simulink model "canTransceiverModel"  (R2018a)
settings: Solver=FixedStepDiscrete  StartTime=0.0  StopTime=50  RelTol=1e-3  EnableMultiTasking=on
values from neighbouring files (symbols this model uses):
  sampleTime = 0.040    (= 0.04)    [canTrasceiverConfig.m]
  sensorLocationConfig = uint8(sensorLocationConfig)    [canTrasceiverConfig.m]
undefined symbols (not defined in the file or in its folder): canChannel, CRC
libraries: simulink x81, canmsglib x27, canlib x8, commcrc2 x1
(part 2 of 5)

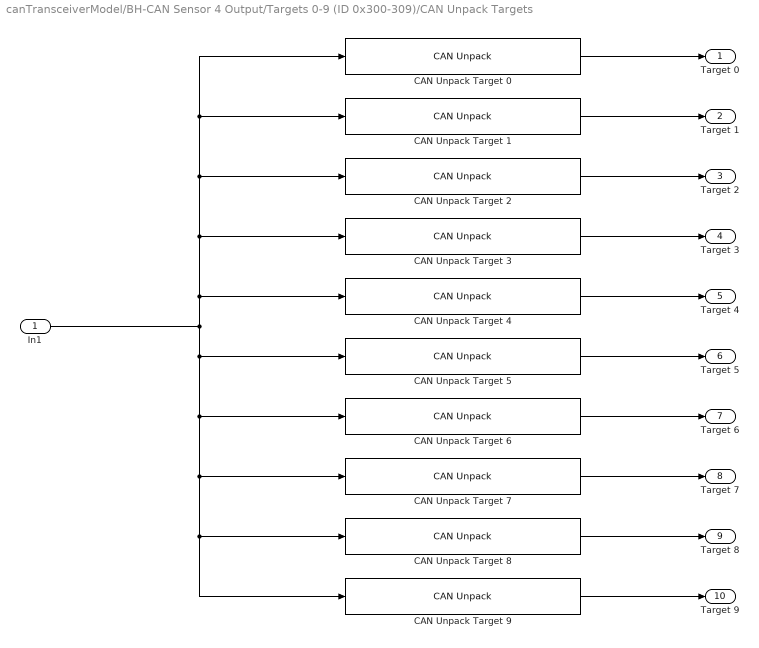
== system canTransceiverModel/BH-CAN Sensor 4 Output/Targets 0-9 (ID 0x300-309)/CAN Unpack Targets ==
  In1 : Inport
  CAN Unpack Target 0 : canmsglib/CAN Unpack  CANdbFile=VehicleInfo.dbc  MsgList=WheelSpeeds  MsgName=Target 0  MsgIDType=Standard (11-bit identifier)  MsgIdentifier=hex2dec('300')  MsgLength=8  SignalInfo=LF_WSpeed$8$16$2$2$1$0$1.000000e-02$-100$0$2000$#LR_WSpeed$40$16$2$2$1$0$1.000000e-02$-100$0$2000$#RF_WSpeed$24$16$2$2$1$0$1.000000e-02$-100$0$2000$#RR_WSpeed$56$16$2$2$1$0$1.000000e-02$-100$0$2000$#  NSignals=4  IDPort=off  TimestampPort=off  ErrorPort=off  RemotePort=off  LengthPort=off  StatusPort=off  StartBits=str2num('[int32(8);int32(40);int32(24);int32(56)]')  SignalSizes=str2num('[int32(16);int32(16);int32(16);int32(16)]')  ByteOrders=str2num('[int32(2);int32(2);int32(2);int32(2)]')  DataTypes=str2num('[int32(2);int32(2);int32(2);int32(2)]')  MultiplexTypes=str2num('[int32(1);int32(1);int32(1);int32(1)]')  MultiplexValues=str2num('[double(0);double(0);double(0);double(0)]')  Factors=str2num('[double(1.000000e-02);double(1.000000e-02);double(1.000000e-02);double(1.000000e-02)]')  Offsets=str2num('[double(-100);double(-100);double(-100);double(-100)]')  Minimums=str2num('[double(0);double(0);double(0);double(0)]')  Maximums=str2num('[double(2000);double(2000);double(2000);double(2000)]')  ApplyMinMax=off
      settings: SourceProductName=Simulink Real-Time  SourceProductBaseCode=XP  DataFormat=raw data
  CAN Unpack Target 1 : canmsglib/CAN Unpack  CANdbFile=VehicleInfo.dbc  MsgList=WheelSpeeds  MsgName=Target 1  MsgIDType=Standard (11-bit identifier)  MsgIdentifier=hex2dec('301')  MsgLength=8  SignalInfo=LF_WSpeed$8$16$2$2$1$0$1.000000e-02$-100$0$2000$#LR_WSpeed$40$16$2$2$1$0$1.000000e-02$-100$0$2000$#RF_WSpeed$24$16$2$2$1$0$1.000000e-02$-100$0$2000$#RR_WSpeed$56$16$2$2$1$0$1.000000e-02$-100$0$2000$#  NSignals=4  IDPort=off  TimestampPort=off  ErrorPort=off  RemotePort=off  LengthPort=off  StatusPort=off  StartBits=str2num('[int32(8);int32(40);int32(24);int32(56)]')  SignalSizes=str2num('[int32(16);int32(16);int32(16);int32(16)]')  ByteOrders=str2num('[int32(2);int32(2);int32(2);int32(2)]')  DataTypes=str2num('[int32(2);int32(2);int32(2);int32(2)]')  MultiplexTypes=str2num('[int32(1);int32(1);int32(1);int32(1)]')  MultiplexValues=str2num('[double(0);double(0);double(0);double(0)]')  Factors=str2num('[double(1.000000e-02);double(1.000000e-02);double(1.000000e-02);double(1.000000e-02)]')  Offsets=str2num('[double(-100);double(-100);double(-100);double(-100)]')  Minimums=str2num('[double(0);double(0);double(0);double(0)]')  Maximums=str2num('[double(2000);double(2000);double(2000);double(2000)]')  ApplyMinMax=off
      settings: SourceProductName=Simulink Real-Time  SourceProductBaseCode=XP  DataFormat=raw data
  CAN Unpack Target 2 : canmsglib/CAN Unpack  CANdbFile=VehicleInfo.dbc  MsgList=WheelSpeeds  MsgName=Target 2  MsgIDType=Standard (11-bit identifier)  MsgIdentifier=hex2dec('302')  MsgLength=8  SignalInfo=LF_WSpeed$8$16$2$2$1$0$1.000000e-02$-100$0$2000$#LR_WSpeed$40$16$2$2$1$0$1.000000e-02$-100$0$2000$#RF_WSpeed$24$16$2$2$1$0$1.000000e-02$-100$0$2000$#RR_WSpeed$56$16$2$2$1$0$1.000000e-02$-100$0$2000$#  NSignals=4  IDPort=off  TimestampPort=off  ErrorPort=off  RemotePort=off  LengthPort=off  StatusPort=off  StartBits=str2num('[int32(8);int32(40);int32(24);int32(56)]')  SignalSizes=str2num('[int32(16);int32(16);int32(16);int32(16)]')  ByteOrders=str2num('[int32(2);int32(2);int32(2);int32(2)]')  DataTypes=str2num('[int32(2);int32(2);int32(2);int32(2)]')  MultiplexTypes=str2num('[int32(1);int32(1);int32(1);int32(1)]')  MultiplexValues=str2num('[double(0);double(0);double(0);double(0)]')  Factors=str2num('[double(1.000000e-02);double(1.000000e-02);double(1.000000e-02);double(1.000000e-02)]')  Offsets=str2num('[double(-100);double(-100);double(-100);double(-100)]')  Minimums=str2num('[double(0);double(0);double(0);double(0)]')  Maximums=str2num('[double(2000);double(2000);double(2000);double(2000)]')  ApplyMinMax=off
      settings: SourceProductName=Simulink Real-Time  SourceProductBaseCode=XP  DataFormat=raw data
  CAN Unpack Target 3 : canmsglib/CAN Unpack  CANdbFile=VehicleInfo.dbc  MsgList=WheelSpeeds  MsgName=Target 3  MsgIDType=Standard (11-bit identifier)  MsgIdentifier=hex2dec('303')  MsgLength=8  SignalInfo=LF_WSpeed$8$16$2$2$1$0$1.000000e-02$-100$0$2000$#LR_WSpeed$40$16$2$2$1$0$1.000000e-02$-100$0$2000$#RF_WSpeed$24$16$2$2$1$0$1.000000e-02$-100$0$2000$#RR_WSpeed$56$16$2$2$1$0$1.000000e-02$-100$0$2000$#  NSignals=4  IDPort=off  TimestampPort=off  ErrorPort=off  RemotePort=off  LengthPort=off  StatusPort=off  StartBits=str2num('[int32(8);int32(40);int32(24);int32(56)]')  SignalSizes=str2num('[int32(16);int32(16);int32(16);int32(16)]')  ByteOrders=str2num('[int32(2);int32(2);int32(2);int32(2)]')  DataTypes=str2num('[int32(2);int32(2);int32(2);int32(2)]')  MultiplexTypes=str2num('[int32(1);int32(1);int32(1);int32(1)]')  MultiplexValues=str2num('[double(0);double(0);double(0);double(0)]')  Factors=str2num('[double(1.000000e-02);double(1.000000e-02);double(1.000000e-02);double(1.000000e-02)]')  Offsets=str2num('[double(-100);double(-100);double(-100);double(-100)]')  Minimums=str2num('[double(0);double(0);double(0);double(0)]')  Maximums=str2num('[double(2000);double(2000);double(2000);double(2000)]')  ApplyMinMax=off
      settings: SourceProductName=Simulink Real-Time  SourceProductBaseCode=XP  DataFormat=raw data
  CAN Unpack Target 4 : canmsglib/CAN Unpack  CANdbFile=VehicleInfo.dbc  MsgList=WheelSpeeds  MsgName=Target 4  MsgIDType=Standard (11-bit identifier)  MsgIdentifier=hex2dec('304')  MsgLength=8  SignalInfo=LF_WSpeed$8$16$2$2$1$0$1.000000e-02$-100$0$2000$#LR_WSpeed$40$16$2$2$1$0$1.000000e-02$-100$0$2000$#RF_WSpeed$24$16$2$2$1$0$1.000000e-02$-100$0$2000$#RR_WSpeed$56$16$2$2$1$0$1.000000e-02$-100$0$2000$#  NSignals=4  IDPort=off  TimestampPort=off  ErrorPort=off  RemotePort=off  LengthPort=off  StatusPort=off  StartBits=str2num('[int32(8);int32(40);int32(24);int32(56)]')  SignalSizes=str2num('[int32(16);int32(16);int32(16);int32(16)]')  ByteOrders=str2num('[int32(2);int32(2);int32(2);int32(2)]')  DataTypes=str2num('[int32(2);int32(2);int32(2);int32(2)]')  MultiplexTypes=str2num('[int32(1);int32(1);int32(1);int32(1)]')  MultiplexValues=str2num('[double(0);double(0);double(0);double(0)]')  Factors=str2num('[double(1.000000e-02);double(1.000000e-02);double(1.000000e-02);double(1.000000e-02)]')  Offsets=str2num('[double(-100);double(-100);double(-100);double(-100)]')  Minimums=str2num('[double(0);double(0);double(0);double(0)]')  Maximums=str2num('[double(2000);double(2000);double(2000);double(2000)]')  ApplyMinMax=off
      settings: SourceProductName=Simulink Real-Time  SourceProductBaseCode=XP  DataFormat=raw data
  CAN Unpack Target 5 : canmsglib/CAN Unpack  CANdbFile=VehicleInfo.dbc  MsgList=WheelSpeeds  MsgName=Target 5  MsgIDType=Standard (11-bit identifier)  MsgIdentifier=hex2dec('305')  MsgLength=8  SignalInfo=LF_WSpeed$8$16$2$2$1$0$1.000000e-02$-100$0$2000$#LR_WSpeed$40$16$2$2$1$0$1.000000e-02$-100$0$2000$#RF_WSpeed$24$16$2$2$1$0$1.000000e-02$-100$0$2000$#RR_WSpeed$56$16$2$2$1$0$1.000000e-02$-100$0$2000$#  NSignals=4  IDPort=off  TimestampPort=off  ErrorPort=off  RemotePort=off  LengthPort=off  StatusPort=off  StartBits=str2num('[int32(8);int32(40);int32(24);int32(56)]')  SignalSizes=str2num('[int32(16);int32(16);int32(16);int32(16)]')  ByteOrders=str2num('[int32(2);int32(2);int32(2);int32(2)]')  DataTypes=str2num('[int32(2);int32(2);int32(2);int32(2)]')  MultiplexTypes=str2num('[int32(1);int32(1);int32(1);int32(1)]')  MultiplexValues=str2num('[double(0);double(0);double(0);double(0)]')  Factors=str2num('[double(1.000000e-02);double(1.000000e-02);double(1.000000e-02);double(1.000000e-02)]')  Offsets=str2num('[double(-100);double(-100);double(-100);double(-100)]')  Minimums=str2num('[double(0);double(0);double(0);double(0)]')  Maximums=str2num('[double(2000);double(2000);double(2000);double(2000)]')  ApplyMinMax=off
      settings: SourceProductName=Simulink Real-Time  SourceProductBaseCode=XP  DataFormat=raw data
  CAN Unpack Target 6 : canmsglib/CAN Unpack  CANdbFile=VehicleInfo.dbc  MsgList=WheelSpeeds  MsgName=Target 6  MsgIDType=Standard (11-bit identifier)  MsgIdentifier=hex2dec('306')  MsgLength=8  SignalInfo=LF_WSpeed$8$16$2$2$1$0$1.000000e-02$-100$0$2000$#LR_WSpeed$40$16$2$2$1$0$1.000000e-02$-100$0$2000$#RF_WSpeed$24$16$2$2$1$0$1.000000e-02$-100$0$2000$#RR_WSpeed$56$16$2$2$1$0$1.000000e-02$-100$0$2000$#  NSignals=4  IDPort=off  TimestampPort=off  ErrorPort=off  RemotePort=off  LengthPort=off  StatusPort=off  StartBits=str2num('[int32(8);int32(40);int32(24);int32(56)]')  SignalSizes=str2num('[int32(16);int32(16);int32(16);int32(16)]')  ByteOrders=str2num('[int32(2);int32(2);int32(2);int32(2)]')  DataTypes=str2num('[int32(2);int32(2);int32(2);int32(2)]')  MultiplexTypes=str2num('[int32(1);int32(1);int32(1);int32(1)]')  MultiplexValues=str2num('[double(0);double(0);double(0);double(0)]')  Factors=str2num('[double(1.000000e-02);double(1.000000e-02);double(1.000000e-02);double(1.000000e-02)]')  Offsets=str2num('[double(-100);double(-100);double(-100);double(-100)]')  Minimums=str2num('[double(0);double(0);double(0);double(0)]')  Maximums=str2num('[double(2000);double(2000);double(2000);double(2000)]')  ApplyMinMax=off
      settings: SourceProductName=Simulink Real-Time  SourceProductBaseCode=XP  DataFormat=raw data
  CAN Unpack Target 7 : canmsglib/CAN Unpack  CANdbFile=VehicleInfo.dbc  MsgList=WheelSpeeds  MsgName=Target 7  MsgIDType=Standard (11-bit identifier)  MsgIdentifier=hex2dec('307')  MsgLength=8  SignalInfo=LF_WSpeed$8$16$2$2$1$0$1.000000e-02$-100$0$2000$#LR_WSpeed$40$16$2$2$1$0$1.000000e-02$-100$0$2000$#RF_WSpeed$24$16$2$2$1$0$1.000000e-02$-100$0$2000$#RR_WSpeed$56$16$2$2$1$0$1.000000e-02$-100$0$2000$#  NSignals=4  IDPort=off  TimestampPort=off  ErrorPort=off  RemotePort=off  LengthPort=off  StatusPort=off  StartBits=str2num('[int32(8);int32(40);int32(24);int32(56)]')  SignalSizes=str2num('[int32(16);int32(16);int32(16);int32(16)]')  ByteOrders=str2num('[int32(2);int32(2);int32(2);int32(2)]')  DataTypes=str2num('[int32(2);int32(2);int32(2);int32(2)]')  MultiplexTypes=str2num('[int32(1);int32(1);int32(1);int32(1)]')  MultiplexValues=str2num('[double(0);double(0);double(0);double(0)]')  Factors=str2num('[double(1.000000e-02);double(1.000000e-02);double(1.000000e-02);double(1.000000e-02)]')  Offsets=str2num('[double(-100);double(-100);double(-100);double(-100)]')  Minimums=str2num('[double(0);double(0);double(0);double(0)]')  Maximums=str2num('[double(2000);double(2000);double(2000);double(2000)]')  ApplyMinMax=off
      settings: SourceProductName=Simulink Real-Time  SourceProductBaseCode=XP  DataFormat=raw data
  CAN Unpack Target 8 : canmsglib/CAN Unpack  CANdbFile=VehicleInfo.dbc  MsgList=WheelSpeeds  MsgName=Target 8  MsgIDType=Standard (11-bit identifier)  MsgIdentifier=hex2dec('308')  MsgLength=8  SignalInfo=LF_WSpeed$8$16$2$2$1$0$1.000000e-02$-100$0$2000$#LR_WSpeed$40$16$2$2$1$0$1.000000e-02$-100$0$2000$#RF_WSpeed$24$16$2$2$1$0$1.000000e-02$-100$0$2000$#RR_WSpeed$56$16$2$2$1$0$1.000000e-02$-100$0$2000$#  NSignals=4  IDPort=off  TimestampPort=off  ErrorPort=off  RemotePort=off  LengthPort=off  StatusPort=off  StartBits=str2num('[int32(8);int32(40);int32(24);int32(56)]')  SignalSizes=str2num('[int32(16);int32(16);int32(16);int32(16)]')  ByteOrders=str2num('[int32(2);int32(2);int32(2);int32(2)]')  DataTypes=str2num('[int32(2);int32(2);int32(2);int32(2)]')  MultiplexTypes=str2num('[int32(1);int32(1);int32(1);int32(1)]')  MultiplexValues=str2num('[double(0);double(0);double(0);double(0)]')  Factors=str2num('[double(1.000000e-02);double(1.000000e-02);double(1.000000e-02);double(1.000000e-02)]')  Offsets=str2num('[double(-100);double(-100);double(-100);double(-100)]')  Minimums=str2num('[double(0);double(0);double(0);double(0)]')  Maximums=str2num('[double(2000);double(2000);double(2000);double(2000)]')  ApplyMinMax=off
      settings: SourceProductName=Simulink Real-Time  SourceProductBaseCode=XP  DataFormat=raw data
  CAN Unpack Target 9 : canmsglib/CAN Unpack  CANdbFile=VehicleInfo.dbc  MsgList=WheelSpeeds  MsgName=Target 9  MsgIDType=Standard (11-bit identifier)  MsgIdentifier=hex2dec('309')  MsgLength=8  SignalInfo=LF_WSpeed$8$16$2$2$1$0$1.000000e-02$-100$0$2000$#LR_WSpeed$40$16$2$2$1$0$1.000000e-02$-100$0$2000$#RF_WSpeed$24$16$2$2$1$0$1.000000e-02$-100$0$2000$#RR_WSpeed$56$16$2$2$1$0$1.000000e-02$-100$0$2000$#  NSignals=4  IDPort=off  TimestampPort=off  ErrorPort=off  RemotePort=off  LengthPort=off  StatusPort=off  StartBits=str2num('[int32(8);int32(40);int32(24);int32(56)]')  SignalSizes=str2num('[int32(16);int32(16);int32(16);int32(16)]')  ByteOrders=str2num('[int32(2);int32(2);int32(2);int32(2)]')  DataTypes=str2num('[int32(2);int32(2);int32(2);int32(2)]')  MultiplexTypes=str2num('[int32(1);int32(1);int32(1);int32(1)]')  MultiplexValues=str2num('[double(0);double(0);double(0);double(0)]')  Factors=str2num('[double(1.000000e-02);double(1.000000e-02);double(1.000000e-02);double(1.000000e-02)]')  Offsets=str2num('[double(-100);double(-100);double(-100);double(-100)]')  Minimums=str2num('[double(0);double(0);double(0);double(0)]')  Maximums=str2num('[double(2000);double(2000);double(2000);double(2000)]')  ApplyMinMax=off
      settings: SourceProductName=Simulink Real-Time  SourceProductBaseCode=XP  DataFormat=raw data
  Target 0 : Outport
  Target 1 : Outport  Port=2
  Target 2 : Outport  Port=3
  Target 3 : Outport  Port=4
  Target 4 : Outport  Port=5
  Target 5 : Outport  Port=6
  Target 6 : Outport  Port=7
  Target 7 : Outport  Port=8
  Target 8 : Outport  Port=9
  Target 9 : Outport  Port=10
  wires:
  In1/1 -> CAN Unpack Target 0/1, CAN Unpack Target 1/1, CAN Unpack Target 2/1, CAN Unpack Target 3/1, CAN Unpack Target 4/1, CAN Unpack Target 9/1, CAN Unpack Target 8/1, CAN Unpack Target 7/1, CAN Unpack Target 6/1, CAN Unpack Target 5/1
  CAN Unpack Target 3/1 -> Target 3/1
  CAN Unpack Target 8/1 -> Target 8/1
  CAN Unpack Target 2/1 -> Target 2/1
  CAN Unpack Target 1/1 -> Target 1/1
  CAN Unpack Target 4/1 -> Target 4/1
  CAN Unpack Target 5/1 -> Target 5/1
  CAN Unpack Target 7/1 -> Target 7/1
  CAN Unpack Target 6/1 -> Target 6/1
  CAN Unpack Target 0/1 -> Target 0/1
  CAN Unpack Target 9/1 -> Target 9/1

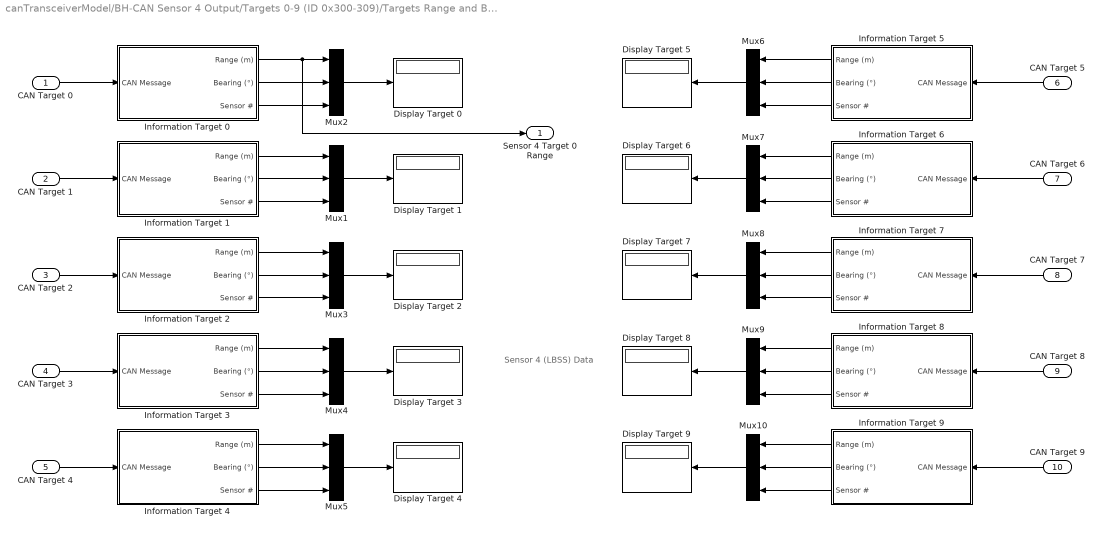
== system canTransceiverModel/BH-CAN Sensor 4 Output/Targets 0-9 (ID 0x300-309)/Targets Range and Bearing Information ==
  note: Sensor 4
      | (LBSS)
      | Data
  CAN Target 0 : Inport
  CAN Target 1 : Inport  Port=2
  CAN Target 2 : Inport  Port=3
  CAN Target 3 : Inport  Port=4
  CAN Target 4 : Inport  Port=5
  CAN Target 5 : Inport  Port=6
  CAN Target 6 : Inport  Port=7
  CAN Target 7 : Inport  Port=8
  CAN Target 8 : Inport  Port=9
  CAN Target 9 : Inport  Port=10
  Display Target {0..9} (10 alike) : Display
  Information Target 0 : Subsystem
  Information Target 1 : Subsystem
  Information Target 2 : Subsystem
  Information Target 3 : Subsystem
  Information Target 4 : Subsystem
  Information Target 5 : Subsystem
  Information Target 6 : Subsystem
  Information Target 7 : Subsystem
  Information Target 8 : Subsystem
  Information Target 9 : Subsystem
  Mux{1..10} (10 alike) : Mux  Inputs=3
  Sensor 4 Target 0 Range : Outport
  wires:
  Information Target 0/2(Bearing (°)) -> Mux2/2
  CAN Target 0/1 -> Information Target 0/1(CAN Message)
  Information Target 0/3(Sensor #) -> Mux2/3
  CAN Target 1/1 -> Information Target 1/1(CAN Message)
  Information Target 1/1(Range (m)) -> Mux1/1
  Information Target 1/3(Sensor #) -> Mux1/3
  Information Target 1/2(Bearing (°)) -> Mux1/2
  CAN Target 2/1 -> Information Target 2/1(CAN Message)
  Information Target 2/1(Range (m)) -> Mux3/1
  Information Target 2/3(Sensor #) -> Mux3/3
  Information Target 2/2(Bearing (°)) -> Mux3/2
  CAN Target 3/1 -> Information Target 3/1(CAN Message)
  Information Target 3/1(Range (m)) -> Mux4/1
  Information Target 3/3(Sensor #) -> Mux4/3
  Information Target 3/2(Bearing (°)) -> Mux4/2
  CAN Target 4/1 -> Information Target 4/1(CAN Message)
  Information Target 4/1(Range (m)) -> Mux5/1
  Information Target 4/3(Sensor #) -> Mux5/3
  Mux5/1 -> Display Target 4/1
  Information Target 4/2(Bearing (°)) -> Mux5/2
  CAN Target 5/1 -> Information Target 5/1(CAN Message)
  Information Target 5/1(Range (m)) -> Mux6/1
  Information Target 5/3(Sensor #) -> Mux6/3
  Mux6/1 -> Display Target 5/1
  Information Target 5/2(Bearing (°)) -> Mux6/2
  Information Target 6/2(Bearing (°)) -> Mux7/2
  Mux7/1 -> Display Target 6/1
  Information Target 6/3(Sensor #) -> Mux7/3
  CAN Target 6/1 -> Information Target 6/1(CAN Message)
  Information Target 6/1(Range (m)) -> Mux7/1
  Information Target 7/2(Bearing (°)) -> Mux8/2
  Mux8/1 -> Display Target 7/1
  Information Target 7/3(Sensor #) -> Mux8/3
  CAN Target 7/1 -> Information Target 7/1(CAN Message)
  Information Target 7/1(Range (m)) -> Mux8/1
  Information Target 8/2(Bearing (°)) -> Mux9/2
  Mux9/1 -> Display Target 8/1
  Information Target 8/3(Sensor #) -> Mux9/3
  CAN Target 8/1 -> Information Target 8/1(CAN Message)
  Information Target 8/1(Range (m)) -> Mux9/1
  Information Target 9/2(Bearing (°)) -> Mux10/2
  Mux10/1 -> Display Target 9/1
  Information Target 9/3(Sensor #) -> Mux10/3
  CAN Target 9/1 -> Information Target 9/1(CAN Message)
  Information Target 9/1(Range (m)) -> Mux10/1
  Mux2/1 -> Display Target 0/1
  Mux4/1 -> Display Target 3/1
  Mux1/1 -> Display Target 1/1
  Mux3/1 -> Display Target 2/1
  Information Target 0/1(Range (m)) -> Sensor 4 Target 0 Range/1, Mux2/1

== system canTransceiverModel/BH-CAN Sensor 3 Output/Targets 0-9 (ID 0x300-309)/Targets Range and Bearing Information/Information Target 0 ==
  CAN Message : Inport
  Check Target Format : Subsystem
  Target Format 2 : Subsystem
  Terminator : Terminator
  Terminator1 : Terminator
  Range (m) : Outport
  Bearing (°) : Outport  Port=2
  Sensor # : Outport  Port=3
  wires:
  Target Format 2/2(Bearing (°)) -> Bearing (°)/1
  CAN Message/1 -> Check Target Format/1(CAN Message), Target Format 2/1(CAN Message)
  Check Target Format/1(Is format 2?) -> Target Format 2/Enable
  Check Target Format/2(Is format 6?) -> Terminator1/1
  Target Format 2/1(Range (m)) -> Range (m)/1
  Target Format 2/3(Sensor #) -> Sensor #/1
  Check Target Format/3(Is neither 2 nor 6?) -> Terminator/1

== system canTransceiverModel/BH-CAN Sensor 3 Output/Targets 0-9 (ID 0x300-309)/Targets Range and Bearing Information/Information Target 1 ==
  CAN Message : Inport
  Check Target Format : Subsystem
  Target Format 2 : Subsystem
  Terminator : Terminator
  Terminator1 : Terminator
  Range (m) : Outport
  Bearing (°) : Outport  Port=2
  Sensor # : Outport  Port=3
  wires:
  Target Format 2/2(Bearing (°)) -> Bearing (°)/1
  CAN Message/1 -> Check Target Format/1(CAN Message), Target Format 2/1(CAN Message)
  Target Format 2/1(Range (m)) -> Range (m)/1
  Target Format 2/3(Sensor #) -> Sensor #/1
  Check Target Format/1(Is format 2?) -> Target Format 2/Enable
  Check Target Format/2(Is format 6?) -> Terminator/1
  Check Target Format/3(Is neither 2 nor 6?) -> Terminator1/1

== system canTransceiverModel/BH-CAN Sensor 3 Output/Targets 0-9 (ID 0x300-309)/Targets Range and Bearing Information/Information Target 2 ==
  CAN Message : Inport
  Check Target Format : Subsystem
  Target Format 2 : Subsystem
  Terminator : Terminator
  Terminator1 : Terminator
  Range (m) : Outport
  Bearing (°) : Outport  Port=2
  Sensor # : Outport  Port=3
  wires:
  Target Format 2/2(Bearing (°)) -> Bearing (°)/1
  CAN Message/1 -> Check Target Format/1(CAN Message), Target Format 2/1(CAN Message)
  Target Format 2/1(Range (m)) -> Range (m)/1
  Target Format 2/3(Sensor #) -> Sensor #/1
  Check Target Format/1(Is format 2?) -> Target Format 2/Enable
  Check Target Format/3(Is neither 2 nor 6?) -> Terminator1/1
  Check Target Format/2(Is format 6?) -> Terminator/1

== system canTransceiverModel/BH-CAN Sensor 3 Output/Targets 0-9 (ID 0x300-309)/Targets Range and Bearing Information/Information Target 3 ==
  CAN Message : Inport
  Check Target Format : Subsystem
  Target Format 2 : Subsystem
  Terminator : Terminator
  Terminator1 : Terminator
  Range (m) : Outport
  Bearing (°) : Outport  Port=2
  Sensor # : Outport  Port=3
  wires:
  Target Format 2/2(Bearing (°)) -> Bearing (°)/1
  CAN Message/1 -> Check Target Format/1(CAN Message), Target Format 2/1(CAN Message)
  Target Format 2/1(Range (m)) -> Range (m)/1
  Target Format 2/3(Sensor #) -> Sensor #/1
  Check Target Format/1(Is format 2?) -> Target Format 2/Enable
  Check Target Format/2(Is format 6?) -> Terminator/1
  Check Target Format/3(Is neither 2 nor 6?) -> Terminator1/1

== system canTransceiverModel/BH-CAN Sensor 3 Output/Targets 0-9 (ID 0x300-309)/Targets Range and Bearing Information/Information Target 4 ==
  CAN Message : Inport
  Check Target Format1 : Subsystem
  Target Format 2 : Subsystem
  Terminator : Terminator
  Terminator1 : Terminator
  Range (m) : Outport
  Bearing (°) : Outport  Port=2
  Sensor # : Outport  Port=3
  wires:
  Target Format 2/2(Bearing (°)) -> Bearing (°)/1
  CAN Message/1 -> Check Target Format1/1(CAN Message), Target Format 2/1(CAN Message)
  Target Format 2/1(Range (m)) -> Range (m)/1
  Target Format 2/3(Sensor #) -> Sensor #/1
  Check Target Format1/1(Is format 2?) -> Target Format 2/Enable
  Check Target Format1/2(Is format 6?) -> Terminator/1
  Check Target Format1/3(Is neither 2 nor 6?) -> Terminator1/1

== system canTransceiverModel/BH-CAN Sensor 3 Output/Targets 0-9 (ID 0x300-309)/Targets Range and Bearing Information/Information Target 5 ==
  CAN Message : Inport
  Check Target Format1 : Subsystem
  Target Format 2 : Subsystem
  Terminator : Terminator
  Terminator1 : Terminator
  Range (m) : Outport
  Bearing (°) : Outport  Port=2
  Sensor # : Outport  Port=3
  wires:
  Target Format 2/2(Bearing (°)) -> Bearing (°)/1
  CAN Message/1 -> Check Target Format1/1(CAN Message), Target Format 2/1(CAN Message)
  Target Format 2/1(Range (m)) -> Range (m)/1
  Target Format 2/3(Sensor #) -> Sensor #/1
  Check Target Format1/1(Is format 2?) -> Target Format 2/Enable
  Check Target Format1/2(Is format 6?) -> Terminator/1
  Check Target Format1/3(Is neither 2 nor 6?) -> Terminator1/1

== system canTransceiverModel/BH-CAN Sensor 3 Output/Targets 0-9 (ID 0x300-309)/Targets Range and Bearing Information/Information Target 6 ==
  CAN Message : Inport
  Check Target Format : Subsystem
  Target Format 2 : Subsystem
  Terminator : Terminator
  Terminator1 : Terminator
  Range (m) : Outport
  Bearing (°) : Outport  Port=2
  Sensor # : Outport  Port=3
  wires:
  Target Format 2/2(Bearing (°)) -> Bearing (°)/1
  CAN Message/1 -> Check Target Format/1(CAN Message), Target Format 2/1(CAN Message)
  Target Format 2/1(Range (m)) -> Range (m)/1
  Target Format 2/3(Sensor #) -> Sensor #/1
  Check Target Format/1(Is format 2?) -> Target Format 2/Enable
  Check Target Format/2(Is format 6?) -> Terminator/1
  Check Target Format/3(Is neither 2 nor 6?) -> Terminator1/1

== system canTransceiverModel/BH-CAN Sensor 3 Output/Targets 0-9 (ID 0x300-309)/Targets Range and Bearing Information/Information Target 7 ==
  CAN Message : Inport
  Check Target Format : Subsystem
  Target Format 2 : Subsystem
  Terminator : Terminator
  Terminator1 : Terminator
  Range (m) : Outport
  Bearing (°) : Outport  Port=2
  Sensor # : Outport  Port=3
  wires:
  Target Format 2/2(Bearing (°)) -> Bearing (°)/1
  CAN Message/1 -> Check Target Format/1(CAN Message), Target Format 2/1(CAN Message)
  Target Format 2/1(Range (m)) -> Range (m)/1
  Target Format 2/3(Sensor #) -> Sensor #/1
  Check Target Format/1(Is format 2?) -> Target Format 2/Enable
  Check Target Format/2(Is format 6?) -> Terminator/1
  Check Target Format/3(Is neither 2 nor 6?) -> Terminator1/1

== system canTransceiverModel/BH-CAN Sensor 3 Output/Targets 0-9 (ID 0x300-309)/Targets Range and Bearing Information/Information Target 8 ==
  CAN Message : Inport
  Check Target Format : Subsystem
  Target Format 2 : Subsystem
  Terminator : Terminator
  Terminator1 : Terminator
  Range (m) : Outport
  Bearing (°) : Outport  Port=2
  Sensor # : Outport  Port=3
  wires:
  Target Format 2/2(Bearing (°)) -> Bearing (°)/1
  CAN Message/1 -> Check Target Format/1(CAN Message), Target Format 2/1(CAN Message)
  Target Format 2/1(Range (m)) -> Range (m)/1
  Target Format 2/3(Sensor #) -> Sensor #/1
  Check Target Format/1(Is format 2?) -> Target Format 2/Enable
  Check Target Format/2(Is format 6?) -> Terminator/1
  Check Target Format/3(Is neither 2 nor 6?) -> Terminator1/1

== system canTransceiverModel/BH-CAN Sensor 3 Output/Targets 0-9 (ID 0x300-309)/Targets Range and Bearing Information/Information Target 9 ==
  CAN Message : Inport
  Check Target Format : Subsystem
  Target Format 2 : Subsystem
  Terminator : Terminator
  Terminator1 : Terminator
  Range (m) : Outport
  Bearing (°) : Outport  Port=2
  Sensor # : Outport  Port=3
  wires:
  Target Format 2/2(Bearing (°)) -> Bearing (°)/1
  CAN Message/1 -> Check Target Format/1(CAN Message), Target Format 2/1(CAN Message)
  Target Format 2/1(Range (m)) -> Range (m)/1
  Target Format 2/3(Sensor #) -> Sensor #/1
  Check Target Format/1(Is format 2?) -> Target Format 2/Enable
  Check Target Format/2(Is format 6?) -> Terminator/1
  Check Target Format/3(Is neither 2 nor 6?) -> Terminator1/1

== system canTransceiverModel/BH-CAN Sensor 4 Output/Targets 0-9 (ID 0x300-309)/Targets Range and Bearing Information/Information Target 0 ==
  CAN Message : Inport
  Check Target Format : Subsystem
  Target Format 2 : Subsystem
  Terminator : Terminator
  Terminator1 : Terminator
  Range (m) : Outport
  Bearing (°) : Outport  Port=2
  Sensor # : Outport  Port=3
  wires:
  Target Format 2/2(Bearing (°)) -> Bearing (°)/1
  CAN Message/1 -> Check Target Format/1(CAN Message), Target Format 2/1(CAN Message)
  Target Format 2/1(Range (m)) -> Range (m)/1
  Target Format 2/3(Sensor #) -> Sensor #/1
  Check Target Format/1(Is format 2?) -> Target Format 2/Enable
  Check Target Format/2(Is format 6?) -> Terminator/1
  Check Target Format/3(Is neither 2 nor 6?) -> Terminator1/1

== system canTransceiverModel/BH-CAN Sensor 4 Output/Targets 0-9 (ID 0x300-309)/Targets Range and Bearing Information/Information Target 1 ==
  CAN Message : Inport
  Check Target Format : Subsystem
  Target Format 2 : Subsystem
  Terminator : Terminator
  Terminator1 : Terminator
  Range (m) : Outport
  Bearing (°) : Outport  Port=2
  Sensor # : Outport  Port=3
  wires:
  Target Format 2/2(Bearing (°)) -> Bearing (°)/1
  Target Format 2/1(Range (m)) -> Range (m)/1
  Target Format 2/3(Sensor #) -> Sensor #/1
  Check Target Format/1(Is format 2?) -> Target Format 2/Enable
  Check Target Format/2(Is format 6?) -> Terminator/1
  Check Target Format/3(Is neither 2 nor 6?) -> Terminator1/1
  CAN Message/1 -> Check Target Format/1(CAN Message), Target Format 2/1(CAN Message)

== system canTransceiverModel/BH-CAN Sensor 4 Output/Targets 0-9 (ID 0x300-309)/Targets Range and Bearing Information/Information Target 2 ==
  CAN Message : Inport
  Check Target Format : Subsystem
  Target Format 2 : Subsystem
  Terminator : Terminator
  Terminator1 : Terminator
  Range (m) : Outport
  Bearing (°) : Outport  Port=2
  Sensor # : Outport  Port=3
  wires:
  Target Format 2/2(Bearing (°)) -> Bearing (°)/1
  Target Format 2/1(Range (m)) -> Range (m)/1
  Target Format 2/3(Sensor #) -> Sensor #/1
  CAN Message/1 -> Check Target Format/1(CAN Message), Target Format 2/1(CAN Message)
  Check Target Format/2(Is format 6?) -> Terminator/1
  Check Target Format/3(Is neither 2 nor 6?) -> Terminator1/1
  Check Target Format/1(Is format 2?) -> Target Format 2/Enable

== system canTransceiverModel/BH-CAN Sensor 4 Output/Targets 0-9 (ID 0x300-309)/Targets Range and Bearing Information/Information Target 3 ==
  CAN Message : Inport
  Check Target Format : Subsystem
  Target Format 2 : Subsystem
  Terminator : Terminator
  Terminator1 : Terminator
  Range (m) : Outport
  Bearing (°) : Outport  Port=2
  Sensor # : Outport  Port=3
  wires:
  Target Format 2/2(Bearing (°)) -> Bearing (°)/1
  Target Format 2/1(Range (m)) -> Range (m)/1
  Target Format 2/3(Sensor #) -> Sensor #/1
  CAN Message/1 -> Check Target Format/1(CAN Message), Target Format 2/1(CAN Message)
  Check Target Format/2(Is format 6?) -> Terminator/1
  Check Target Format/3(Is neither 2 nor 6?) -> Terminator1/1
  Check Target Format/1(Is format 2?) -> Target Format 2/Enable

== system canTransceiverModel/BH-CAN Sensor 4 Output/Targets 0-9 (ID 0x300-309)/Targets Range and Bearing Information/Information Target 4 ==
  CAN Message : Inport
  Check Target Format : Subsystem
  Target Format 2 : Subsystem
  Terminator : Terminator
  Terminator1 : Terminator
  Range (m) : Outport
  Bearing (°) : Outport  Port=2
  Sensor # : Outport  Port=3
  wires:
  Target Format 2/2(Bearing (°)) -> Bearing (°)/1
  Target Format 2/1(Range (m)) -> Range (m)/1
  Target Format 2/3(Sensor #) -> Sensor #/1
  CAN Message/1 -> Check Target Format/1(CAN Message), Target Format 2/1(CAN Message)
  Check Target Format/2(Is format 6?) -> Terminator/1
  Check Target Format/3(Is neither 2 nor 6?) -> Terminator1/1
  Check Target Format/1(Is format 2?) -> Target Format 2/Enable

== system canTransceiverModel/BH-CAN Sensor 4 Output/Targets 0-9 (ID 0x300-309)/Targets Range and Bearing Information/Information Target 5 ==
  CAN Message : Inport
  Check Target Format : Subsystem
  Target Format 2 : Subsystem
  Terminator : Terminator
  Terminator1 : Terminator
  Range (m) : Outport
  Bearing (°) : Outport  Port=2
  Sensor # : Outport  Port=3
  wires:
  Target Format 2/2(Bearing (°)) -> Bearing (°)/1
  Target Format 2/1(Range (m)) -> Range (m)/1
  Target Format 2/3(Sensor #) -> Sensor #/1
  CAN Message/1 -> Check Target Format/1(CAN Message), Target Format 2/1(CAN Message)
  Check Target Format/2(Is format 6?) -> Terminator/1
  Check Target Format/3(Is neither 2 nor 6?) -> Terminator1/1
  Check Target Format/1(Is format 2?) -> Target Format 2/Enable

== system canTransceiverModel/BH-CAN Sensor 4 Output/Targets 0-9 (ID 0x300-309)/Targets Range and Bearing Information/Information Target 6 ==
  CAN Message : Inport
  Check Target Format : Subsystem
  Target Format 2 : Subsystem
  Terminator : Terminator
  Terminator1 : Terminator
  Range (m) : Outport
  Bearing (°) : Outport  Port=2
  Sensor # : Outport  Port=3
  wires:
  Target Format 2/2(Bearing (°)) -> Bearing (°)/1
  Target Format 2/1(Range (m)) -> Range (m)/1
  Target Format 2/3(Sensor #) -> Sensor #/1
  CAN Message/1 -> Check Target Format/1(CAN Message), Target Format 2/1(CAN Message)
  Check Target Format/2(Is format 6?) -> Terminator/1
  Check Target Format/3(Is neither 2 nor 6?) -> Terminator1/1
  Check Target Format/1(Is format 2?) -> Target Format 2/Enable

== system canTransceiverModel/BH-CAN Sensor 4 Output/Targets 0-9 (ID 0x300-309)/Targets Range and Bearing Information/Information Target 7 ==
  CAN Message : Inport
  Check Target Format : Subsystem
  Target Format 2 : Subsystem
  Terminator : Terminator
  Terminator1 : Terminator
  Range (m) : Outport
  Bearing (°) : Outport  Port=2
  Sensor # : Outport  Port=3
  wires:
  Target Format 2/2(Bearing (°)) -> Bearing (°)/1
  Target Format 2/1(Range (m)) -> Range (m)/1
  Target Format 2/3(Sensor #) -> Sensor #/1
  CAN Message/1 -> Check Target Format/1(CAN Message), Target Format 2/1(CAN Message)
  Check Target Format/2(Is format 6?) -> Terminator/1
  Check Target Format/3(Is neither 2 nor 6?) -> Terminator1/1
  Check Target Format/1(Is format 2?) -> Target Format 2/Enable

== system canTransceiverModel/BH-CAN Sensor 4 Output/Targets 0-9 (ID 0x300-309)/Targets Range and Bearing Information/Information Target 8 ==
  CAN Message : Inport
  Check Target Format : Subsystem
  Target Format 2 : Subsystem
  Terminator : Terminator
  Terminator1 : Terminator
  Range (m) : Outport
  Bearing (°) : Outport  Port=2
  Sensor # : Outport  Port=3
  wires:
  Target Format 2/2(Bearing (°)) -> Bearing (°)/1
  Target Format 2/1(Range (m)) -> Range (m)/1
  Target Format 2/3(Sensor #) -> Sensor #/1
  CAN Message/1 -> Check Target Format/1(CAN Message), Target Format 2/1(CAN Message)
  Check Target Format/2(Is format 6?) -> Terminator/1
  Check Target Format/3(Is neither 2 nor 6?) -> Terminator1/1
  Check Target Format/1(Is format 2?) -> Target Format 2/Enable

== system canTransceiverModel/BH-CAN Sensor 4 Output/Targets 0-9 (ID 0x300-309)/Targets Range and Bearing Information/Information Target 9 ==
  CAN Message : Inport
  Check Target Format : Subsystem
  Target Format 2 : Subsystem
  Terminator : Terminator
  Terminator1 : Terminator
  Range (m) : Outport
  Bearing (°) : Outport  Port=2
  Sensor # : Outport  Port=3
  wires:
  Target Format 2/2(Bearing (°)) -> Bearing (°)/1
  Target Format 2/1(Range (m)) -> Range (m)/1
  Target Format 2/3(Sensor #) -> Sensor #/1
  CAN Message/1 -> Check Target Format/1(CAN Message), Target Format 2/1(CAN Message)
  Check Target Format/2(Is format 6?) -> Terminator/1
  Check Target Format/3(Is neither 2 nor 6?) -> Terminator1/1
  Check Target Format/1(Is format 2?) -> Target Format 2/Enable

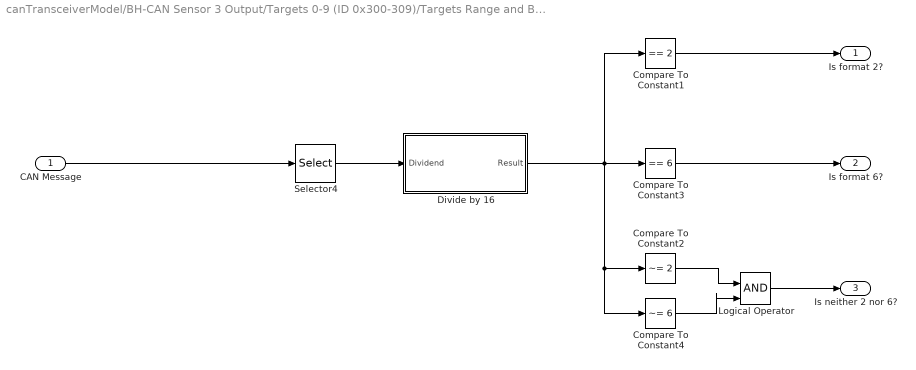
== system canTransceiverModel/BH-CAN Sensor 3 Output/Targets 0-9 (ID 0x300-309)/Targets Range and Bearing Information/Information Target 0/Check Target Format ==
  CAN Message : Inport
  Compare To Constant1 : simulink/Logic and Bit Operations/Compare To Constant  relop===  const=2  OutDataTypeStr=boolean
  Compare To Constant2 : simulink/Logic and Bit Operations/Compare To Constant  relop=~=  const=2  OutDataTypeStr=boolean
  Compare To Constant3 : simulink/Logic and Bit Operations/Compare To Constant  relop===  const=6  OutDataTypeStr=boolean
  Compare To Constant4 : simulink/Logic and Bit Operations/Compare To Constant  relop=~=  const=6  OutDataTypeStr=boolean
  Divide by 16 : Subsystem
  Logical Operator : Logic  IconShape=distinctive  AllPortsSameDT=off  OutDataTypeStr=boolean
  Selector4 : Selector  IndexMode=Zero-based  InputPortWidth=8  IndexOptions=Index vector (dialog)  Indices=6  OutputSizes=1
  Is format 2? : Outport
  Is format 6? : Outport  Port=2
  Is neither 2 nor 6? : Outport  Port=3
  wires:
  CAN Message/1 -> Selector4/1
  Selector4/1 -> Divide by 16/1(Dividend)
  Compare To Constant1/1 -> Is format 2?/1
  Compare To Constant3/1 -> Is format 6?/1
  Compare To Constant2/1 -> Logical Operator/1
  Divide by 16/1(Result) -> Compare To Constant4/1, Compare To Constant2/1, Compare To Constant3/1, Compare To Constant1/1
  Compare To Constant4/1 -> Logical Operator/2
  Logical Operator/1 -> Is neither 2 nor 6?/1

== system canTransceiverModel/BH-CAN Sensor 3 Output/Targets 0-9 (ID 0x300-309)/Targets Range and Bearing Information/Information Target 0/Target Format 2 ==
  CAN Message : Inport
  Enable : EnablePort
  Bearing : Subsystem
  Range : Subsystem
  Sensor number : Subsystem
  Range (m) : Outport
  Bearing (°) : Outport  Port=2
  Sensor # : Outport  Port=3
  wires:
  CAN Message/1 -> Sensor number/1(CAN Message), Bearing/1(CAN Message), Range/1(CAN Message)
  Range/1(Range (m)) -> Range (m)/1
  Bearing/1(Bearing (°)) -> Bearing (°)/1
  Sensor number/1(Sensor #) -> Sensor #/1

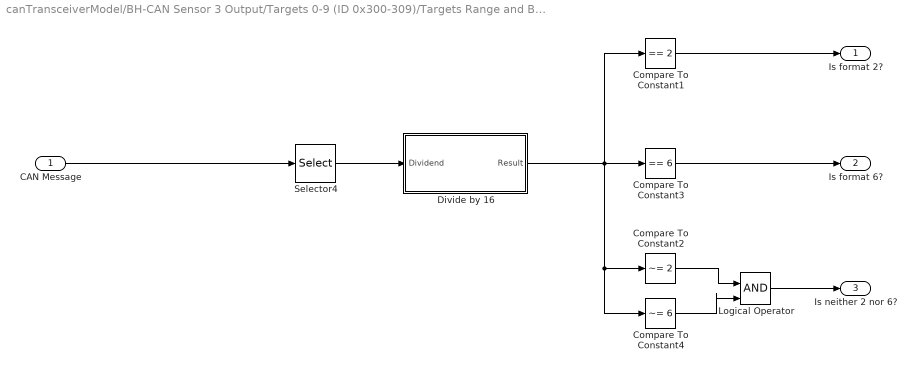
== system canTransceiverModel/BH-CAN Sensor 3 Output/Targets 0-9 (ID 0x300-309)/Targets Range and Bearing Information/Information Target 1/Check Target Format ==
  CAN Message : Inport
  Compare To Constant1 : simulink/Logic and Bit Operations/Compare To Constant  relop===  const=2  OutDataTypeStr=boolean
  Compare To Constant2 : simulink/Logic and Bit Operations/Compare To Constant  relop=~=  const=2  OutDataTypeStr=boolean
  Compare To Constant3 : simulink/Logic and Bit Operations/Compare To Constant  relop===  const=6  OutDataTypeStr=boolean
  Compare To Constant4 : simulink/Logic and Bit Operations/Compare To Constant  relop=~=  const=6  OutDataTypeStr=boolean
  Divide by 16 : Subsystem
  Logical Operator : Logic  IconShape=distinctive  AllPortsSameDT=off  OutDataTypeStr=boolean
  Selector4 : Selector  IndexMode=Zero-based  InputPortWidth=8  IndexOptions=Index vector (dialog)  Indices=6  OutputSizes=1
  Is format 2? : Outport
  Is format 6? : Outport  Port=2
  Is neither 2 nor 6? : Outport  Port=3
  wires:
  CAN Message/1 -> Selector4/1
  Selector4/1 -> Divide by 16/1(Dividend)
  Compare To Constant1/1 -> Is format 2?/1
  Compare To Constant3/1 -> Is format 6?/1
  Compare To Constant2/1 -> Logical Operator/1
  Divide by 16/1(Result) -> Compare To Constant4/1, Compare To Constant2/1, Compare To Constant3/1, Compare To Constant1/1
  Compare To Constant4/1 -> Logical Operator/2
  Logical Operator/1 -> Is neither 2 nor 6?/1

== system canTransceiverModel/BH-CAN Sensor 3 Output/Targets 0-9 (ID 0x300-309)/Targets Range and Bearing Information/Information Target 1/Target Format 2 ==
  CAN Message : Inport
  Enable : EnablePort
  Bearing : Subsystem
  Range : Subsystem
  Sensor number : Subsystem
  Range (m) : Outport
  Bearing (°) : Outport  Port=2
  Sensor # : Outport  Port=3
  wires:
  CAN Message/1 -> Sensor number/1(CAN Message), Bearing/1(CAN Message), Range/1(CAN Message)
  Range/1(Range (m)) -> Range (m)/1
  Bearing/1(Bearing (°)) -> Bearing (°)/1
  Sensor number/1(Sensor #) -> Sensor #/1

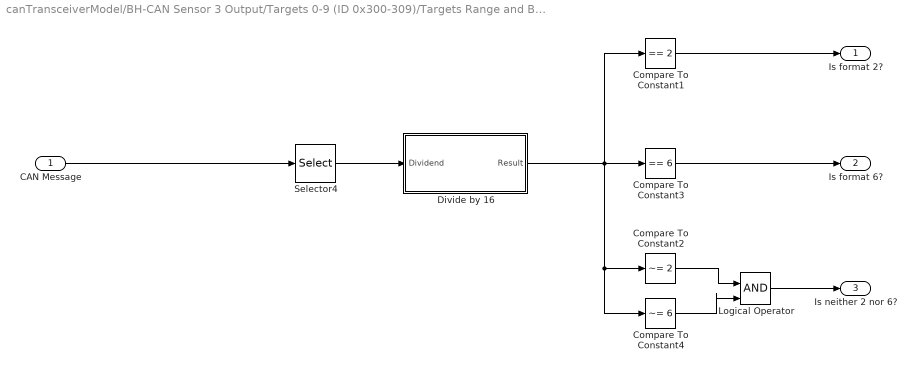
== system canTransceiverModel/BH-CAN Sensor 3 Output/Targets 0-9 (ID 0x300-309)/Targets Range and Bearing Information/Information Target 2/Check Target Format ==
  CAN Message : Inport
  Compare To Constant1 : simulink/Logic and Bit Operations/Compare To Constant  relop===  const=2  OutDataTypeStr=boolean
  Compare To Constant2 : simulink/Logic and Bit Operations/Compare To Constant  relop=~=  const=2  OutDataTypeStr=boolean
  Compare To Constant3 : simulink/Logic and Bit Operations/Compare To Constant  relop===  const=6  OutDataTypeStr=boolean
  Compare To Constant4 : simulink/Logic and Bit Operations/Compare To Constant  relop=~=  const=6  OutDataTypeStr=boolean
  Divide by 16 : Subsystem
  Logical Operator : Logic  IconShape=distinctive  AllPortsSameDT=off  OutDataTypeStr=boolean
  Selector4 : Selector  IndexMode=Zero-based  InputPortWidth=8  IndexOptions=Index vector (dialog)  Indices=6  OutputSizes=1
  Is format 2? : Outport
  Is format 6? : Outport  Port=2
  Is neither 2 nor 6? : Outport  Port=3
  wires:
  CAN Message/1 -> Selector4/1
  Selector4/1 -> Divide by 16/1(Dividend)
  Compare To Constant1/1 -> Is format 2?/1
  Compare To Constant3/1 -> Is format 6?/1
  Compare To Constant2/1 -> Logical Operator/1
  Divide by 16/1(Result) -> Compare To Constant4/1, Compare To Constant2/1, Compare To Constant3/1, Compare To Constant1/1
  Compare To Constant4/1 -> Logical Operator/2
  Logical Operator/1 -> Is neither 2 nor 6?/1

== system canTransceiverModel/BH-CAN Sensor 3 Output/Targets 0-9 (ID 0x300-309)/Targets Range and Bearing Information/Information Target 2/Target Format 2 ==
  CAN Message : Inport
  Enable : EnablePort
  Bearing : Subsystem
  Range : Subsystem
  Sensor number : Subsystem
  Range (m) : Outport
  Bearing (°) : Outport  Port=2
  Sensor # : Outport  Port=3
  wires:
  CAN Message/1 -> Sensor number/1(CAN Message), Bearing/1(CAN Message), Range/1(CAN Message)
  Range/1(Range (m)) -> Range (m)/1
  Bearing/1(Bearing (°)) -> Bearing (°)/1
  Sensor number/1(Sensor #) -> Sensor #/1

== system canTransceiverModel/BH-CAN Sensor 3 Output/Targets 0-9 (ID 0x300-309)/Targets Range and Bearing Information/Information Target 3/Check Target Format ==
  CAN Message : Inport
  Compare To Constant1 : simulink/Logic and Bit Operations/Compare To Constant  relop===  const=2  OutDataTypeStr=boolean
  Compare To Constant2 : simulink/Logic and Bit Operations/Compare To Constant  relop=~=  const=2  OutDataTypeStr=boolean
  Compare To Constant3 : simulink/Logic and Bit Operations/Compare To Constant  relop===  const=6  OutDataTypeStr=boolean
  Compare To Constant4 : simulink/Logic and Bit Operations/Compare To Constant  relop=~=  const=6  OutDataTypeStr=boolean
  Divide by 16 : Subsystem
  Logical Operator : Logic  IconShape=distinctive  AllPortsSameDT=off  OutDataTypeStr=boolean
  Selector4 : Selector  IndexMode=Zero-based  InputPortWidth=8  IndexOptions=Index vector (dialog)  Indices=6  OutputSizes=1
  Is format 2? : Outport
  Is format 6? : Outport  Port=2
  Is neither 2 nor 6? : Outport  Port=3
  wires:
  CAN Message/1 -> Selector4/1
  Selector4/1 -> Divide by 16/1(Dividend)
  Compare To Constant1/1 -> Is format 2?/1
  Compare To Constant3/1 -> Is format 6?/1
  Compare To Constant2/1 -> Logical Operator/1
  Divide by 16/1(Result) -> Compare To Constant4/1, Compare To Constant2/1, Compare To Constant3/1, Compare To Constant1/1
  Compare To Constant4/1 -> Logical Operator/2
  Logical Operator/1 -> Is neither 2 nor 6?/1

== system canTransceiverModel/BH-CAN Sensor 3 Output/Targets 0-9 (ID 0x300-309)/Targets Range and Bearing Information/Information Target 3/Target Format 2 ==
  CAN Message : Inport
  Enable : EnablePort
  Bearing : Subsystem
  Range : Subsystem
  Sensor number : Subsystem
  Range (m) : Outport
  Bearing (°) : Outport  Port=2
  Sensor # : Outport  Port=3
  wires:
  CAN Message/1 -> Sensor number/1(CAN Message), Bearing/1(CAN Message), Range/1(CAN Message)
  Range/1(Range (m)) -> Range (m)/1
  Bearing/1(Bearing (°)) -> Bearing (°)/1
  Sensor number/1(Sensor #) -> Sensor #/1

== system canTransceiverModel/BH-CAN Sensor 3 Output/Targets 0-9 (ID 0x300-309)/Targets Range and Bearing Information/Information Target 4/Check Target Format1 ==
  CAN Message : Inport
  Compare To Constant1 : simulink/Logic and Bit Operations/Compare To Constant  relop===  const=2  OutDataTypeStr=boolean
  Compare To Constant2 : simulink/Logic and Bit Operations/Compare To Constant  relop=~=  const=2  OutDataTypeStr=boolean
  Compare To Constant3 : simulink/Logic and Bit Operations/Compare To Constant  relop===  const=6  OutDataTypeStr=boolean
  Compare To Constant4 : simulink/Logic and Bit Operations/Compare To Constant  relop=~=  const=6  OutDataTypeStr=boolean
  Divide by 16 : Subsystem
  Logical Operator : Logic  IconShape=distinctive  AllPortsSameDT=off  OutDataTypeStr=boolean
  Selector4 : Selector  IndexMode=Zero-based  InputPortWidth=8  IndexOptions=Index vector (dialog)  Indices=6  OutputSizes=1
  Is format 2? : Outport
  Is format 6? : Outport  Port=2
  Is neither 2 nor 6? : Outport  Port=3
  wires:
  CAN Message/1 -> Selector4/1
  Selector4/1 -> Divide by 16/1(Dividend)
  Compare To Constant1/1 -> Is format 2?/1
  Compare To Constant3/1 -> Is format 6?/1
  Compare To Constant2/1 -> Logical Operator/1
  Divide by 16/1(Result) -> Compare To Constant4/1, Compare To Constant2/1, Compare To Constant3/1, Compare To Constant1/1
  Compare To Constant4/1 -> Logical Operator/2
  Logical Operator/1 -> Is neither 2 nor 6?/1

== system canTransceiverModel/BH-CAN Sensor 3 Output/Targets 0-9 (ID 0x300-309)/Targets Range and Bearing Information/Information Target 4/Target Format 2 ==
  CAN Message : Inport
  Enable : EnablePort
  Bearing : Subsystem
  Range : Subsystem
  Sensor number : Subsystem
  Range (m) : Outport
  Bearing (°) : Outport  Port=2
  Sensor # : Outport  Port=3
  wires:
  CAN Message/1 -> Sensor number/1(CAN Message), Bearing/1(CAN Message), Range/1(CAN Message)
  Range/1(Range (m)) -> Range (m)/1
  Bearing/1(Bearing (°)) -> Bearing (°)/1
  Sensor number/1(Sensor #) -> Sensor #/1

== system canTransceiverModel/BH-CAN Sensor 3 Output/Targets 0-9 (ID 0x300-309)/Targets Range and Bearing Information/Information Target 5/Check Target Format1 ==
  CAN Message : Inport
  Compare To Constant1 : simulink/Logic and Bit Operations/Compare To Constant  relop===  const=2  OutDataTypeStr=boolean
  Compare To Constant2 : simulink/Logic and Bit Operations/Compare To Constant  relop=~=  const=2  OutDataTypeStr=boolean
  Compare To Constant3 : simulink/Logic and Bit Operations/Compare To Constant  relop===  const=6  OutDataTypeStr=boolean
  Compare To Constant4 : simulink/Logic and Bit Operations/Compare To Constant  relop=~=  const=6  OutDataTypeStr=boolean
  Divide by 16 : Subsystem
  Logical Operator : Logic  IconShape=distinctive  AllPortsSameDT=off  OutDataTypeStr=boolean
  Selector4 : Selector  IndexMode=Zero-based  InputPortWidth=8  IndexOptions=Index vector (dialog)  Indices=6  OutputSizes=1
  Is format 2? : Outport
  Is format 6? : Outport  Port=2
  Is neither 2 nor 6? : Outport  Port=3
  wires:
  CAN Message/1 -> Selector4/1
  Selector4/1 -> Divide by 16/1(Dividend)
  Compare To Constant1/1 -> Is format 2?/1
  Compare To Constant3/1 -> Is format 6?/1
  Compare To Constant2/1 -> Logical Operator/1
  Divide by 16/1(Result) -> Compare To Constant4/1, Compare To Constant2/1, Compare To Constant3/1, Compare To Constant1/1
  Compare To Constant4/1 -> Logical Operator/2
  Logical Operator/1 -> Is neither 2 nor 6?/1

== system canTransceiverModel/BH-CAN Sensor 3 Output/Targets 0-9 (ID 0x300-309)/Targets Range and Bearing Information/Information Target 5/Target Format 2 ==
  CAN Message : Inport
  Enable : EnablePort
  Bearing : Subsystem
  Range : Subsystem
  Sensor number : Subsystem
  Range (m) : Outport
  Bearing (°) : Outport  Port=2
  Sensor # : Outport  Port=3
  wires:
  CAN Message/1 -> Sensor number/1(CAN Message), Bearing/1(CAN Message), Range/1(CAN Message)
  Range/1(Range (m)) -> Range (m)/1
  Bearing/1(Bearing (°)) -> Bearing (°)/1
  Sensor number/1(Sensor #) -> Sensor #/1

== system canTransceiverModel/BH-CAN Sensor 3 Output/Targets 0-9 (ID 0x300-309)/Targets Range and Bearing Information/Information Target 6/Check Target Format ==
  CAN Message : Inport
  Compare To Constant1 : simulink/Logic and Bit Operations/Compare To Constant  relop===  const=2  OutDataTypeStr=boolean
  Compare To Constant2 : simulink/Logic and Bit Operations/Compare To Constant  relop=~=  const=2  OutDataTypeStr=boolean
  Compare To Constant3 : simulink/Logic and Bit Operations/Compare To Constant  relop===  const=6  OutDataTypeStr=boolean
  Compare To Constant4 : simulink/Logic and Bit Operations/Compare To Constant  relop=~=  const=6  OutDataTypeStr=boolean
  Divide by 16 : Subsystem
  Logical Operator : Logic  IconShape=distinctive  AllPortsSameDT=off  OutDataTypeStr=boolean
  Selector4 : Selector  IndexMode=Zero-based  InputPortWidth=8  IndexOptions=Index vector (dialog)  Indices=6  OutputSizes=1
  Is format 2? : Outport
  Is format 6? : Outport  Port=2
  Is neither 2 nor 6? : Outport  Port=3
  wires:
  CAN Message/1 -> Selector4/1
  Selector4/1 -> Divide by 16/1(Dividend)
  Compare To Constant1/1 -> Is format 2?/1
  Compare To Constant3/1 -> Is format 6?/1
  Compare To Constant2/1 -> Logical Operator/1
  Divide by 16/1(Result) -> Compare To Constant4/1, Compare To Constant2/1, Compare To Constant3/1, Compare To Constant1/1
  Compare To Constant4/1 -> Logical Operator/2
  Logical Operator/1 -> Is neither 2 nor 6?/1

== system canTransceiverModel/BH-CAN Sensor 3 Output/Targets 0-9 (ID 0x300-309)/Targets Range and Bearing Information/Information Target 6/Target Format 2 ==
  CAN Message : Inport
  Enable : EnablePort
  Bearing : Subsystem
  Range : Subsystem
  Sensor number : Subsystem
  Range (m) : Outport
  Bearing (°) : Outport  Port=2
  Sensor # : Outport  Port=3
  wires:
  CAN Message/1 -> Sensor number/1(CAN Message), Bearing/1(CAN Message), Range/1(CAN Message)
  Range/1(Range (m)) -> Range (m)/1
  Bearing/1(Bearing (°)) -> Bearing (°)/1
  Sensor number/1(Sensor #) -> Sensor #/1

== system canTransceiverModel/BH-CAN Sensor 3 Output/Targets 0-9 (ID 0x300-309)/Targets Range and Bearing Information/Information Target 7/Check Target Format ==
  CAN Message : Inport
  Compare To Constant1 : simulink/Logic and Bit Operations/Compare To Constant  relop===  const=2  OutDataTypeStr=boolean
  Compare To Constant2 : simulink/Logic and Bit Operations/Compare To Constant  relop=~=  const=2  OutDataTypeStr=boolean
  Compare To Constant3 : simulink/Logic and Bit Operations/Compare To Constant  relop===  const=6  OutDataTypeStr=boolean
  Compare To Constant4 : simulink/Logic and Bit Operations/Compare To Constant  relop=~=  const=6  OutDataTypeStr=boolean
  Divide by 16 : Subsystem
  Logical Operator : Logic  IconShape=distinctive  AllPortsSameDT=off  OutDataTypeStr=boolean
  Selector4 : Selector  IndexMode=Zero-based  InputPortWidth=8  IndexOptions=Index vector (dialog)  Indices=6  OutputSizes=1
  Is format 2? : Outport
  Is format 6? : Outport  Port=2
  Is neither 2 nor 6? : Outport  Port=3
  wires:
  CAN Message/1 -> Selector4/1
  Selector4/1 -> Divide by 16/1(Dividend)
  Compare To Constant1/1 -> Is format 2?/1
  Compare To Constant3/1 -> Is format 6?/1
  Compare To Constant2/1 -> Logical Operator/1
  Divide by 16/1(Result) -> Compare To Constant4/1, Compare To Constant2/1, Compare To Constant3/1, Compare To Constant1/1
  Compare To Constant4/1 -> Logical Operator/2
  Logical Operator/1 -> Is neither 2 nor 6?/1
